simulink model "Block0_m"  (Simulink 7.9)
settings: Solver=ode45  SolverMode=SingleTasking  StartTime=0.0  StopTime=999999  MaxStep=10  RelTol=1e-3  AbsTol=1e-3
values from neighbouring files (symbols this model uses):
  U = st_Varia('LongNames')    [block0_i.m]
  x0 = []    [block0_i.m]    (also in block0_s.m = x0)
undefined symbols (not defined in the file or in its folder): B
settings Model: Creator=M.Sparnaaij  LastModifiedBy=M.Sparnaaij
settings DataIOCC: LimitDataPoints=off  SaveOutput=off  SaveTime=off  SignalLoggingName=sigsOut
settings OptimizationCC: BooleanDataType=off
settings DebuggingCC: SaveWithParameterizedLinksMsg=none  SignalResolutionControl=TryResolveAllWithWarning  SolverPrmCheckMsg=none  MultiTaskDSMMsg=warning  MultiTaskCondExecSysMsg=none  StrictBusMsg=None
settings HardwareCC: TargetUnknown=on
settings RTWCC: IncludeERTFirstTime=on
settings GRTTargetCC: CombineOutputUpdateFcns=off  GRTInterface=on

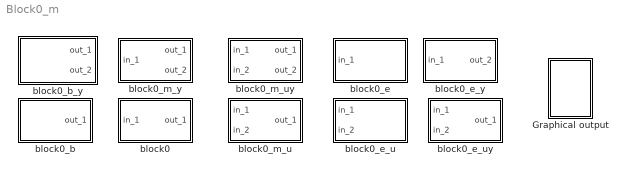
== system Block0_m ==
  Graphical output : Subsystem
      settings: OpenFcn=block0_g
      mask Display:
      | plot(0,0,100,100,[80,20,20],[20,20,80],[80,69,60,52,45,39,33,28,24,20],[65,65,64,61,57,52,45,37,30,20])
      | disp('');
      | text(100,100,'block0', 'horizontalAlignment', 'right', 'verticalAlignment', 'top');
  block0 : Subsystem  Description=block0
      mask init:
      | filenaam='.\StimelaData\block0_p.mat';
      | 
      | [Pn,Fn,Fext]=Fileprop(filenaam);
      | 
      | errstr = st_UniqName(filenaam,'filenaam=''','SubSystem','OpenFcn');
      | if errstr, error([errstr 'The filename "' filenaam '" is already in use. Choose a different filename.']), end
      | 
      | P = block0_p(filenaam);
      | [B,x0,U]=block0_i(filenaam);
      settings: OpenFcn=|
      | filenaam='block0_p.mat';
      | st_ParameterInput('init',gcb,filenaam,'block0');
      mask Display:
      | plot(0,0,100,100,[0 20],[50 50],[0 20],[55 55],[80 100],[ 50 50],[80 100],[ 55 55],[20 80 80 20 20],[10 10 90  90 10]);
      | disp('')
      | text(50,50,'block0', 'horizontalAlignment', 'center', 'verticalAlignment', 'middle');
      | text(50,0,Fn, 'horizontalAlignment', 'center', 'verticalAlignment', 'base');
  block0_b : Subsystem  Description=block0
      mask init: same as Block0_m/block0
      settings: OpenFcn=|
      | filenaam='block0_p.mat';
      | st_ParameterInput('init',gcb,filenaam,'block0');
      mask Display:
      | plot(0,0,100,100,[80 100],[ 50 50],[80 100],[ 55 55],[20 80 80 20 20],[10 10 90  90 10]);
      | disp('')
      | text(50,50,'block0', 'horizontalAlignment', 'center', 'verticalAlignment', 'middle');
      | text(50,0,Fn, 'horizontalAlignment', 'center', 'verticalAlignment', 'base');
  block0_b_y : Subsystem  Description=block0
      mask init:
      | filenaam='.\StimelaData\block0_p.mat';
      | 
      | [Pn,Fn,Fext]=Fileprop(filenaam);
      | 
      | errstr = st_UniqName(filenaam,'filenaam=''','SubSystem','OpenFcn');
      | if errstr, error([errstr 'The filename "' filenaam '" is already in use. Choose a different filename.']), end
      | 
      | P = block0_p(filenaam);
      | [B,x0,U]=block0_i(filenaam);
      settings: OpenFcn=|
      | filenaam='block0_p.mat';
      | st_ParameterInput('init',gcb,filenaam,'block0');
      mask Display:
      | plot(0,0,100,100,[80 100],[80 80],[80 100],[85 85],[80 100],[ 20 20],[20 80 80 20 20],[10 10 90 90 10]);
      | disp('')
      | text(50,50,'block0', 'horizontalAlignment', 'center', 'verticalAlignment', 'middle');
      | text(50,0,Fn, 'horizontalAlignment', 'center', 'verticalAlignment', 'base');
  block0_e : Subsystem  Description=block0
      mask init: same as Block0_m/block0
      settings: OpenFcn=|
      | filenaam='block0_p.mat';
      | st_ParameterInput('init',gcb,filenaam,'block0');
      mask Display:
      | plot(0,0,100,100,[0 20],[ 50 50],[0 20],[ 55 55],[20 80 80 20 20],[10 10 90  90 10]);
      | disp('')
      | text(50,50,'block0', 'horizontalAlignment', 'center', 'verticalAlignment', 'middle');
      | text(50,0,Fn, 'horizontalAlignment', 'center', 'verticalAlignment', 'base');
  block0_e_u : Subsystem  Description=block0
      mask init:
      | filenaam='.\StimelaData\block0_p.mat';
      | 
      | [Pn,Fn,Fext]=Fileprop(filenaam);
      | 
      | errstr = st_UniqName(filenaam,'filenaam=''','SubSystem','OpenFcn');
      | if errstr, error([errstr 'The filename "' filenaam '" is already in use. Choose a different filename.']), end
      | 
      | P = block0_p(filenaam);
      | [B,x0,U]=block0_i(filenaam);
      | V = st_Varia;
      settings: OpenFcn=|
      | filenaam='block0_p.mat';
      | st_ParameterInput('init',gcb,filenaam,'block0');
      mask Display:
      | plot(0,0,100,100,[0 20],[80 80],[0 20],[85 85],[0 20],[20 20],[20 80 80 20 20],[10 10 90  90 10]);
      | disp('')
      | text(50,50,'block0', 'horizontalAlignment', 'center', 'verticalAlignment', 'middle');
      | text(50,0,Fn, 'horizontalAlignment', 'center', 'verticalAlignment', 'base');
  block0_e_uy : Subsystem  Description=block0
      mask init: same as Block0_m/block0_e_u
      settings: OpenFcn=|
      | filenaam='block0_p.mat';
      | st_ParameterInput('init',gcb,filenaam,'block0');
      mask Display:
      | plot(0,0,100,100,[0 20],[80 80],[0 20],[85 85],[0 20],[20 20],[80 100],[ 20 20],[20 80 80 20 20],[10 10 90  90 10]);
      | disp('')
      | text(50,50,'block0', 'horizontalAlignment', 'center', 'verticalAlignment', 'middle');
      | text(50,0,Fn, 'horizontalAlignment', 'center', 'verticalAlignment', 'base');
  block0_e_y : Subsystem  Description=block0
      mask init: same as Block0_m/block0
      settings: OpenFcn=|
      | filenaam='block0_p.mat';
      | st_ParameterInput('init',gcb,filenaam,'block0');
      mask Display:
      | plot(0,0,100,100,[0 20],[50 50],[0 20],[55 55],[80 100],[ 20 20],[20 80 80 20 20],[10 10 90  90 10]);
      | disp('')
      | text(50,50,'block0', 'horizontalAlignment', 'center', 'verticalAlignment', 'middle');
      | text(50,0,Fn, 'horizontalAlignment', 'center', 'verticalAlignment', 'base');
  block0_m_u : Subsystem  Description=block0
      mask init: same as Block0_m/block0_e_u
      settings: OpenFcn=|
      | filenaam='block0_p.mat';
      | st_ParameterInput('init',gcb,filenaam,'block0');
      mask Display:
      | plot(0,0,100,100,[0 20],[85 85],[0 20],[80 80],[0 20],[20 20],[80 100],[ 50 50],[80 100],[ 55 55],[20 80 80 20 20],[10 10 90  90 10]);
      | disp('')
      | text(50,50,'block0', 'horizontalAlignment', 'center', 'verticalAlignment', 'middle');
      | text(50,0,Fn, 'horizontalAlignment', 'center', 'verticalAlignment', 'base');
  block0_m_uy : Subsystem  Description=block0
      mask init: same as Block0_m/block0
      settings: OpenFcn=|
      | filenaam='block0_p.mat';
      | st_ParameterInput('init',gcb,filenaam,'block0');
      mask Display:
      | plot(0,0,100,100,[0 20],[80 80],[0 20],[85 85],[0 20],[20 20],[80 100],[80 80],[80 100],[85 85],[80 100],[ 20 20],[20 80 80 20 20],[10 10 90  90 10]);
      | disp('')
      | text(50,50,'block0', 'horizontalAlignment', 'center', 'verticalAlignment', 'middle');
      | text(50,0,Fn, 'horizontalAlignment', 'center', 'verticalAlignment', 'base');
  block0_m_y : Subsystem  Description=block0
      mask init: same as Block0_m/block0
      settings: OpenFcn=|
      | filenaam='block0_p.mat';
      | st_ParameterInput('init',gcb,filenaam,'block0');
      mask Display:
      | plot(0,0,100,100,[0 20],[50 50],[0 20],[55 55],[80 100],[80 80],[80 100],[85 85],[80 100],[ 20 20],[20 80 80 20 20],[10 10 90  90 10]);
      | disp('')
      | text(50,50,'block0', 'horizontalAlignment', 'center', 'verticalAlignment', 'middle');
      | text(50,0,Fn, 'horizontalAlignment', 'center', 'verticalAlignment', 'base');

== system Block0_m/Graphical output ==
  note: plotten

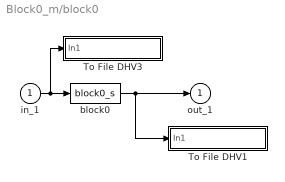
== system Block0_m/block0 ==
  in_1 : Inport
  To File DHV1 : Subsystem  mask(To File DHV){naam=[filenaam(1:length(filenaam)-4) '_out.sti']}
      mask prompts: naam "Naam van bestand"
      mask init:
      | set_param([gcb '/To File'],'Filename',naam);
      mask Display: disp(naam)
  To File DHV3 : Subsystem  mask(To File DHV){naam=[filenaam(1:length(filenaam)-4) '_in.sti']}
      mask prompts: naam "Naam van bestand"
      mask init:
      | set_param([gcb '/To File'],'Filename',naam);
      mask Display: disp(naam)
  block0 : S-Function  FunctionName=block0_s  Parameters=B,x0,U,P  EnableBusSupport=off
  out_1 : Outport  InitialOutput=0
  wires:
  in_1/1 -> block0/1, To File DHV3/1(In1)
  block0/1 -> out_1/1, To File DHV1/1(In1)

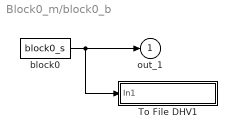
== system Block0_m/block0_b ==
  To File DHV1 : Subsystem  mask(To File DHV){naam=[filenaam(1:length(filenaam)-4) '_out.sti']}
      mask prompts: naam "Naam van bestand"
      mask init:
      | set_param([gcb '/To File'],'Filename',naam);
      mask Display: disp(naam)
  block0 : S-Function  FunctionName=block0_s  Parameters=B,x0,U,P  EnableBusSupport=off
  out_1 : Outport  InitialOutput=0
  wires:
  block0/1 -> out_1/1, To File DHV1/1(In1)

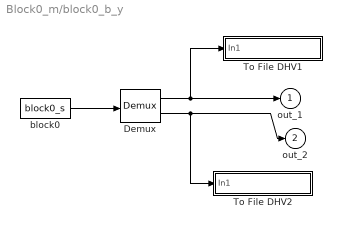
== system Block0_m/block0_b_y ==
  Demux : Demux  Outputs=[U.Number B.Measurements]
  To File DHV1 : Subsystem  mask(To File DHV){naam=[filenaam(1:length(filenaam)-4) '_out.sti']}
      mask prompts: naam "Naam van bestand"
      mask init:
      | set_param([gcb '/To File'],'Filename',naam);
      mask Display: disp(naam)
  To File DHV2 : Subsystem  mask(To File DHV){naam=[filenaam(1:length(filenaam)-4) '_EM.sti']}
      mask prompts: naam "Naam van bestand"
      mask init:
      | set_param([gcb '/To File'],'Filename',naam);
      mask Display: disp(naam)
  block0 : S-Function  FunctionName=block0_s  Parameters=B,x0,U,P  EnableBusSupport=off
  out_1 : Outport  InitialOutput=0
  out_2 : Outport  Port=2  InitialOutput=0
  wires:
  block0/1 -> Demux/1
  Demux/1 -> out_1/1, To File DHV1/1(In1)
  Demux/2 -> out_2/1, To File DHV2/1(In1)

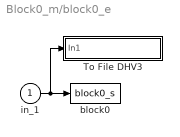
== system Block0_m/block0_e ==
  in_1 : Inport
  To File DHV3 : Subsystem  mask(To File DHV){naam=[filenaam(1:length(filenaam)-4) '_in.sti']}
      mask prompts: naam "Naam van bestand"
      mask init:
      | set_param([gcb '/To File'],'Filename',naam);
      mask Display: disp(naam)
  block0 : S-Function  FunctionName=block0_s  Parameters=B,x0,U,P  EnableBusSupport=off
  wires:
  in_1/1 -> To File DHV3/1(In1), block0/1

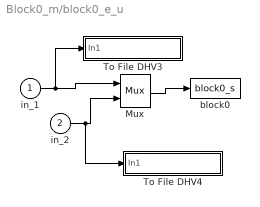
== system Block0_m/block0_e_u ==
  in_1 : Inport
  in_2 : Inport  Port=2
  Mux : Mux  Inputs=[U.Number B.Setpoints]
  To File DHV3 : Subsystem  mask(To File DHV){naam=[filenaam(1:length(filenaam)-4) '_in.sti']}
      mask prompts: naam "Naam van bestand"
      mask init:
      | set_param([gcb '/To File'],'Filename',naam);
      mask Display: disp(naam)
  To File DHV4 : Subsystem  mask(To File DHV){naam=[filenaam(1:length(filenaam)-4) '_ES.sti']}
      mask prompts: naam "Naam van bestand"
      mask init:
      | set_param([gcb '/To File'],'Filename',naam);
      mask Display: disp(naam)
  block0 : S-Function  FunctionName=block0_s  Parameters=B,x0,U,P  EnableBusSupport=off
  wires:
  Mux/1 -> block0/1
  in_1/1 -> Mux/1, To File DHV3/1(In1)
  in_2/1 -> Mux/2, To File DHV4/1(In1)

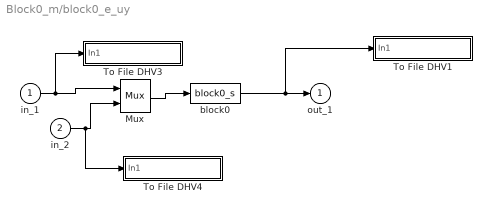
== system Block0_m/block0_e_uy ==
  in_1 : Inport
  in_2 : Inport  Port=2
  Mux : Mux  Inputs=[U.Number B.Setpoints]
  To File DHV1 : Subsystem  mask(To File DHV){naam=[filenaam(1:length(filenaam)-4) '_EM.sti']}
      mask prompts: naam "Naam van bestand"
      mask init:
      | set_param([gcb '/To File'],'Filename',naam);
      mask Display: disp(naam)
  To File DHV3 : Subsystem  mask(To File DHV){naam=[filenaam(1:length(filenaam)-4) '_in.sti']}
      mask prompts: naam "Naam van bestand"
      mask init:
      | set_param([gcb '/To File'],'Filename',naam);
      mask Display: disp(naam)
  To File DHV4 : Subsystem  mask(To File DHV){naam=[filenaam(1:length(filenaam)-4) '_ES.sti']}
      mask prompts: naam "Naam van bestand"
      mask init:
      | set_param([gcb '/To File'],'Filename',naam);
      mask Display: disp(naam)
  block0 : S-Function  FunctionName=block0_s  Parameters=B,x0,U,P  EnableBusSupport=off
  out_1 : Outport  InitialOutput=0
  wires:
  block0/1 -> out_1/1, To File DHV1/1(In1)
  Mux/1 -> block0/1
  in_1/1 -> Mux/1, To File DHV3/1(In1)
  in_2/1 -> Mux/2, To File DHV4/1(In1)

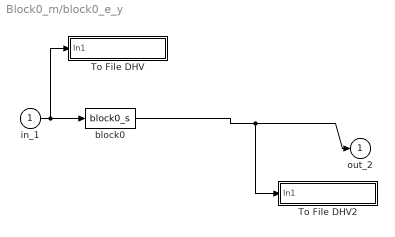
== system Block0_m/block0_e_y ==
  in_1 : Inport
  To File DHV : Subsystem  mask(To File DHV){naam=[filenaam(1:length(filenaam)-4) '_in.sti']}
      mask prompts: naam "Naam van bestand"
      mask init:
      | set_param([gcb '/To File'],'Filename',naam);
      mask Display: disp(naam)
  To File DHV2 : Subsystem  mask(To File DHV){naam=[filenaam(1:length(filenaam)-4) '_EM.sti']}
      mask prompts: naam "Naam van bestand"
      mask init:
      | set_param([gcb '/To File'],'Filename',naam);
      mask Display: disp(naam)
  block0 : S-Function  FunctionName=block0_s  Parameters=B,x0,U,P  EnableBusSupport=off
  out_2 : Outport  InitialOutput=0
  wires:
  block0/1 -> out_2/1, To File DHV2/1(In1)
  in_1/1 -> block0/1, To File DHV/1(In1)

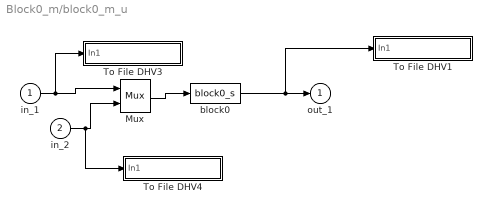
== system Block0_m/block0_m_u ==
  in_1 : Inport
  in_2 : Inport  Port=2
  Mux : Mux  Inputs=[U.Number B.Setpoints]
  To File DHV1 : Subsystem  mask(To File DHV){naam=[filenaam(1:length(filenaam)-4) '_out.sti']}
      mask prompts: naam "Naam van bestand"
      mask init:
      | set_param([gcb '/To File'],'Filename',naam);
      mask Display: disp(naam)
  To File DHV3 : Subsystem  mask(To File DHV){naam=[filenaam(1:length(filenaam)-4) '_in.sti']}
      mask prompts: naam "Naam van bestand"
      mask init:
      | set_param([gcb '/To File'],'Filename',naam);
      mask Display: disp(naam)
  To File DHV4 : Subsystem  mask(To File DHV){naam=[filenaam(1:length(filenaam)-4) '_ES.sti']}
      mask prompts: naam "Naam van bestand"
      mask init:
      | set_param([gcb '/To File'],'Filename',naam);
      mask Display: disp(naam)
  block0 : S-Function  FunctionName=block0_s  Parameters=B,x0,U,P  EnableBusSupport=off
  out_1 : Outport  InitialOutput=0
  wires:
  block0/1 -> out_1/1, To File DHV1/1(In1)
  Mux/1 -> block0/1
  in_1/1 -> Mux/1, To File DHV3/1(In1)
  in_2/1 -> Mux/2, To File DHV4/1(In1)

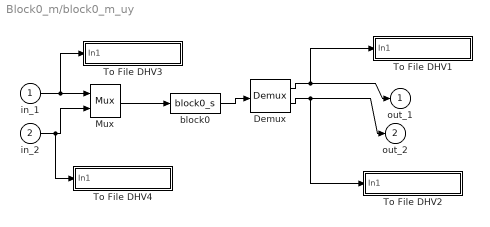
== system Block0_m/block0_m_uy ==
  in_1 : Inport
  in_2 : Inport  Port=2
  Demux : Demux  Outputs=[U.Number B.Measurements]
  Mux : Mux  Inputs=[U.Number B.Setpoints]
  To File DHV1 : Subsystem  mask(To File DHV){naam=[filenaam(1:length(filenaam)-4) '_out.sti']}
      mask prompts: naam "Naam van bestand"
      mask init:
      | set_param([gcb '/To File'],'Filename',naam);
      mask Display: disp(naam)
  To File DHV2 : Subsystem  mask(To File DHV){naam=[filenaam(1:length(filenaam)-4) '_EM.sti']}
      mask prompts: naam "Naam van bestand"
      mask init:
      | set_param([gcb '/To File'],'Filename',naam);
      mask Display: disp(naam)
  To File DHV3 : Subsystem  mask(To File DHV){naam=[filenaam(1:length(filenaam)-4) '_in.sti']}
      mask prompts: naam "Naam van bestand"
      mask init:
      | set_param([gcb '/To File'],'Filename',naam);
      mask Display: disp(naam)
  To File DHV4 : Subsystem  mask(To File DHV){naam=[filenaam(1:length(filenaam)-4) '_ES.sti']}
      mask prompts: naam "Naam van bestand"
      mask init:
      | set_param([gcb '/To File'],'Filename',naam);
      mask Display: disp(naam)
  block0 : S-Function  FunctionName=block0_s  Parameters=B,x0,U,P  EnableBusSupport=off
  out_1 : Outport  InitialOutput=0
  out_2 : Outport  Port=2  InitialOutput=0
  wires:
  Demux/2 -> out_2/1, To File DHV2/1(In1)
  Demux/1 -> out_1/1, To File DHV1/1(In1)
  block0/1 -> Demux/1
  in_1/1 -> Mux/1, To File DHV3/1(In1)
  Mux/1 -> block0/1
  in_2/1 -> Mux/2, To File DHV4/1(In1)

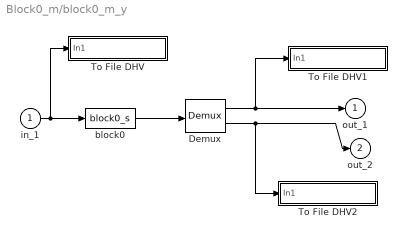
== system Block0_m/block0_m_y ==
  in_1 : Inport
  Demux : Demux  Outputs=[U.Number B.Measurements]
  To File DHV : Subsystem  mask(To File DHV){naam=[filenaam(1:length(filenaam)-4) '_in.sti']}
      mask prompts: naam "Naam van bestand"
      mask init:
      | set_param([gcb '/To File'],'Filename',naam);
      mask Display: disp(naam)
  To File DHV1 : Subsystem  mask(To File DHV){naam=[filenaam(1:length(filenaam)-4) '_out.sti']}
      mask prompts: naam "Naam van bestand"
      mask init:
      | set_param([gcb '/To File'],'Filename',naam);
      mask Display: disp(naam)
  To File DHV2 : Subsystem  mask(To File DHV){naam=[filenaam(1:length(filenaam)-4) '_EM.sti']}
      mask prompts: naam "Naam van bestand"
      mask init:
      | set_param([gcb '/To File'],'Filename',naam);
      mask Display: disp(naam)
  block0 : S-Function  FunctionName=block0_s  Parameters=B,x0,U,P  EnableBusSupport=off
  out_1 : Outport  InitialOutput=0
  out_2 : Outport  Port=2  InitialOutput=0
  wires:
  block0/1 -> Demux/1
  Demux/1 -> out_1/1, To File DHV1/1(In1)
  Demux/2 -> out_2/1, To File DHV2/1(In1)
  in_1/1 -> block0/1, To File DHV/1(In1)

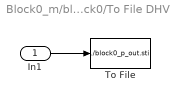
== system Block0_m/block0/To File DHV1 ==
  In1 : Inport
  To File : ToFile  Filename=./block0_p_out.sti  MatrixName=block0out
  wires:
  In1/1 -> To File/1

== system Block0_m/block0/To File DHV3 ==
  In1 : Inport
  To File : ToFile  Filename=./block0_p_in.sti  MatrixName=block0in
  wires:
  In1/1 -> To File/1

== system Block0_m/block0_b/To File DHV1 ==
  In1 : Inport
  To File : ToFile  Filename=./block0_p_out.sti  MatrixName=block0out
  wires:
  In1/1 -> To File/1

== system Block0_m/block0_b_y/To File DHV1 ==
  In1 : Inport
  To File : ToFile  Filename=./block0_p_out.sti  MatrixName=block0out
  wires:
  In1/1 -> To File/1

== system Block0_m/block0_b_y/To File DHV2 ==
  In1 : Inport
  To File : ToFile  Filename=./block0_p_EM.sti  MatrixName=block0EM
  wires:
  In1/1 -> To File/1

== system Block0_m/block0_e/To File DHV3 ==
  In1 : Inport
  To File : ToFile  Filename=./block0_p_in.sti  MatrixName=block0in
  wires:
  In1/1 -> To File/1

== system Block0_m/block0_e_u/To File DHV3 ==
  In1 : Inport
  To File : ToFile  Filename=./block0_p_in.sti  MatrixName=block0in
  wires:
  In1/1 -> To File/1

== system Block0_m/block0_e_u/To File DHV4 ==
  In1 : Inport
  To File : ToFile  Filename=./block0_p_ES.sti  MatrixName=block0ES
  wires:
  In1/1 -> To File/1

== system Block0_m/block0_e_uy/To File DHV1 ==
  In1 : Inport
  To File : ToFile  Filename=./block0_p_EM.sti  MatrixName=block0EM
  wires:
  In1/1 -> To File/1

== system Block0_m/block0_e_uy/To File DHV3 ==
  In1 : Inport
  To File : ToFile  Filename=./block0_p_in.sti  MatrixName=block0in
  wires:
  In1/1 -> To File/1

== system Block0_m/block0_e_uy/To File DHV4 ==
  In1 : Inport
  To File : ToFile  Filename=./block0_p_ES.sti  MatrixName=block0ES
  wires:
  In1/1 -> To File/1

== system Block0_m/block0_e_y/To File DHV ==
  In1 : Inport
  To File : ToFile  Filename=./block0_p_in.sti  MatrixName=block0in
  wires:
  In1/1 -> To File/1

== system Block0_m/block0_e_y/To File DHV2 ==
  In1 : Inport
  To File : ToFile  Filename=./block0_p_EM.sti  MatrixName=block0EM
  wires:
  In1/1 -> To File/1

== system Block0_m/block0_m_u/To File DHV1 ==
  In1 : Inport
  To File : ToFile  Filename=./block0_p_out.sti  MatrixName=block0out
  wires:
  In1/1 -> To File/1

== system Block0_m/block0_m_u/To File DHV3 ==
  In1 : Inport
  To File : ToFile  Filename=./block0_p_in.sti  MatrixName=block0in
  wires:
  In1/1 -> To File/1

== system Block0_m/block0_m_u/To File DHV4 ==
  In1 : Inport
  To File : ToFile  Filename=./block0_p_ES.sti  MatrixName=block0ES
  wires:
  In1/1 -> To File/1

== system Block0_m/block0_m_uy/To File DHV1 ==
  In1 : Inport
  To File : ToFile  Filename=./block0_p_out.sti  MatrixName=block0out
  wires:
  In1/1 -> To File/1

== system Block0_m/block0_m_uy/To File DHV2 ==
  In1 : Inport
  To File : ToFile  Filename=./block0_p_EM.sti  MatrixName=block0EM
  wires:
  In1/1 -> To File/1

== system Block0_m/block0_m_uy/To File DHV3 ==
  In1 : Inport
  To File : ToFile  Filename=./block0_p_in.sti  MatrixName=block0in
  wires:
  In1/1 -> To File/1

== system Block0_m/block0_m_uy/To File DHV4 ==
  In1 : Inport
  To File : ToFile  Filename=./block0_p_ES.sti  MatrixName=block0ES
  wires:
  In1/1 -> To File/1

== system Block0_m/block0_m_y/To File DHV ==
  In1 : Inport
  To File : ToFile  Filename=./block0_p_in.sti  MatrixName=block0in
  wires:
  In1/1 -> To File/1

== system Block0_m/block0_m_y/To File DHV1 ==
  In1 : Inport
  To File : ToFile  Filename=./block0_p_out.sti  MatrixName=block0out
  wires:
  In1/1 -> To File/1

== system Block0_m/block0_m_y/To File DHV2 ==
  In1 : Inport
  To File : ToFile  Filename=./block0_p_EM.sti  MatrixName=block0EM
  wires:
  In1/1 -> To File/1
